simulink model "IEEE39_IBR_FrequencyControl_Fullversion_2021a"  (R2021a)
settings: Solver=VariableStepAuto  StartTime=0.0  StopTime=30  RelTol=1e-3
InitFcn:
  | IEEE39data_FrencyControl_full_Opensource;
undefined symbols (not defined in the file): alpha, c, eps_ps, eps_u, Fref, IBR_data, line, Sbase, t_start_disturbance, t_startcontrol, Vbase
libraries: spsThreePhaseVIMeasurementLib x61, spsThreePhasePISectionLineLib x34, spsControlledVoltageSourceLib x33, spsabctodq0Lib x33, powerlib_extras x27, spsPLL3phLib x26, spsGroundLib x22, spsThreePhaseSeriesRLCBranchLib x22, spsThreePhaseParallelRLCLoadLib x19, pid_lib x14, spsMeanLib x11, spsdq0toabcLib x11
(part 1 of 5)
settings Model: SimulationMode=accelerator  Creator=wangxy  LastModifiedBy=wangxy
settings DebuggingCC: UnconnectedInputMsg=none  UnconnectedOutputMsg=none  UnconnectedLineMsg=none
settings ModelReferenceCC: EnableRefExpFcnMdlSchedulingChecks=off
settings RTWCC: Description=Generic Real-Time Target  GPUComputeCapability=5.0  DLArmComputeVersion=20.02.1

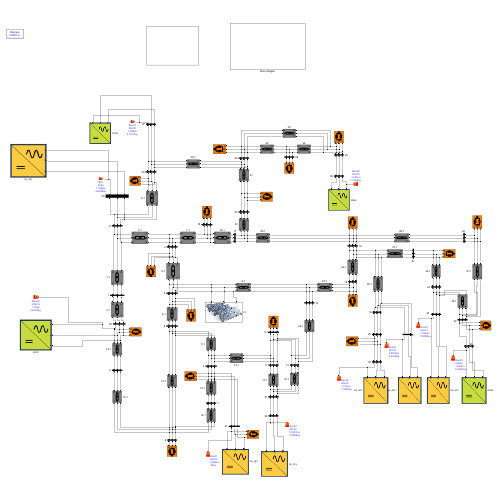
[thumbnail: Simulink's stored preview of the top-level diagram]
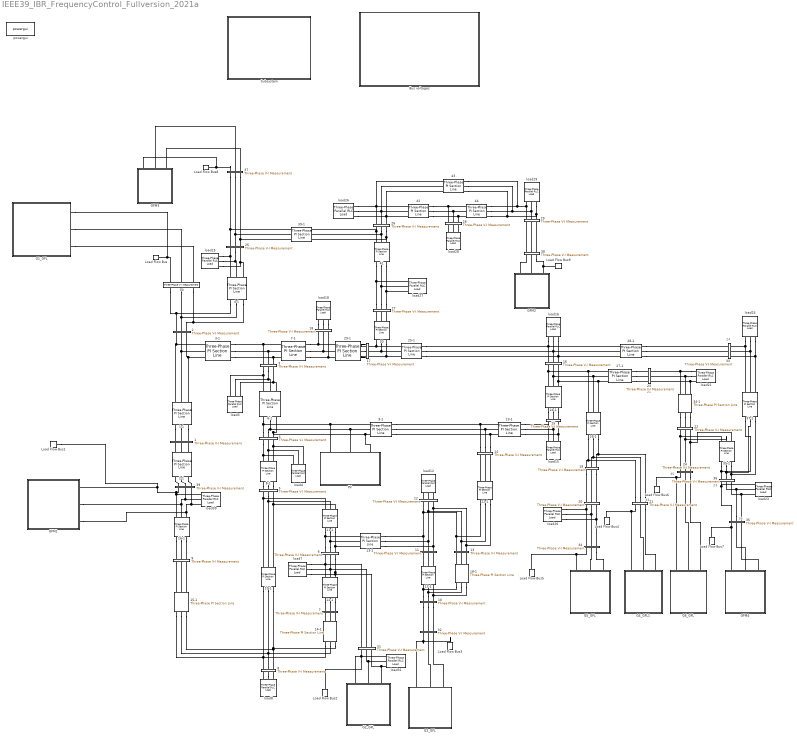
== system IEEE39_IBR_FrequencyControl_Fullversion_2021a ==
  note: 33
  note: 24
  note: 23
  note: 36
  note: 35
  note: 21
  " 30" : spsThreePhasePISectionLineLib/Three-Phase PI Section Line  LConnTagsString=a|b|c  RConnTagsString=A|B|C  Length=1  Frequency=60  Resistances="[line(30,3)  3*line(30,3)]"  Inductances="[line(30,4)  3*line(30,4)]"  Capacitances="[line(30,5)  line(30,5)/3]"
  1 : spsThreePhaseVIMeasurementLib/Three-Phase V-I Measurement  VoltageMeasurement=phase-to-phase  SetLabelV=on  LabelV=Vabc_1  Vpu=off  VpuLL=on  CurrentMeasurement=no  SetLabelI=on  LabelI=Iabc_B2  Ipu=off  Pbase=100e6  Vbase=Bus(1,2)*1e3  OutputType=Complex  PhasorSimulation=off  PSBequivalent=0
  1-1 : spsThreePhasePISectionLineLib/Three-Phase PI Section Line  LConnTagsString=a|b|c  RConnTagsString=A|B|C  Length=1  Frequency=60  Resistances="[line(1,3)  3*line(1,3)]"  Inductances="[line(1,4)  3*line(1,4)]"  Capacitances="[line(1,5)  line(1,5)/3]"
  10 : spsThreePhaseVIMeasurementLib/Three-Phase V-I Measurement  VoltageMeasurement=phase-to-phase  SetLabelV=on  LabelV=Vabc_10  Vpu=off  VpuLL=on  CurrentMeasurement=no  SetLabelI=on  LabelI=Iabc_B2  Ipu=off  Pbase=100e6  Vbase=Bus(10,2)*1e3  OutputType=Complex  PhasorSimulation=off  PSBequivalent=0
  10-1 : spsThreePhasePISectionLineLib/Three-Phase PI Section Line  LConnTagsString=a|b|c  RConnTagsString=A|B|C  Length=1  Frequency=60  Resistances="[line(10,3)  3*line(10,3)]"  Inductances="[line(10,4)  3*line(10,4)]"  Capacitances="[line(10,5)  line(10,5)/3]"
  11 : spsThreePhaseVIMeasurementLib/Three-Phase V-I Measurement  VoltageMeasurement=phase-to-phase  SetLabelV=on  LabelV=Vabc_11  Vpu=off  VpuLL=on  CurrentMeasurement=no  SetLabelI=on  LabelI=Iabc_B2  Ipu=off  Pbase=100e6  Vbase=Bus(11,2)*1e3  OutputType=Complex  PhasorSimulation=off  PSBequivalent=0
  11-1 : spsThreePhasePISectionLineLib/Three-Phase PI Section Line  LConnTagsString=a|b|c  RConnTagsString=A|B|C  Length=1  Frequency=60  Resistances="[line(11,3)  3*line(11,3)]"  Inductances="[line(11,4)  3*line(11,4)]"  Capacitances="[line(11,5)   line(11,5)/3]"
  12 : spsThreePhaseVIMeasurementLib/Three-Phase V-I Measurement  VoltageMeasurement=phase-to-phase  SetLabelV=on  LabelV=Vabc_12  Vpu=off  VpuLL=on  CurrentMeasurement=no  SetLabelI=on  LabelI=Iabc_B2  Ipu=off  Pbase=100e6  Vbase=Bus(12,2)*1e3  OutputType=Complex  PhasorSimulation=off  PSBequivalent=0
  12-1 : spsThreePhasePISectionLineLib/Three-Phase PI Section Line  LConnTagsString=a|b|c  RConnTagsString=A|B|C  Length=1  Frequency=60  Resistances="[line(12,3)  3*line(12,3)]"  Inductances="[line(12,4)  3*line(12,4)]"  Capacitances="[line(12,5)   line(12,5)/3]"
  13 : spsThreePhaseVIMeasurementLib/Three-Phase V-I Measurement  VoltageMeasurement=phase-to-phase  SetLabelV=on  LabelV=Vabc_13  Vpu=off  VpuLL=on  CurrentMeasurement=no  SetLabelI=on  LabelI=Iabc_B2  Ipu=off  Pbase=100e6  Vbase=Bus(13,2)*1e3  OutputType=Complex  PhasorSimulation=off  PSBequivalent=0
  13-1 : spsThreePhasePISectionLineLib/Three-Phase PI Section Line  LConnTagsString=a|b|c  RConnTagsString=A|B|C  Length=1  Frequency=60  Resistances=[line(13,3) 3*line(13,3)]  Inductances="[line(13,4)  3*line(13,4)]"  Capacitances="[line(13,5)  line(13,5)/3]"
  14 : spsThreePhaseVIMeasurementLib/Three-Phase V-I Measurement  VoltageMeasurement=phase-to-phase  SetLabelV=on  LabelV=Vabc_14  Vpu=off  VpuLL=on  CurrentMeasurement=no  SetLabelI=on  LabelI=Iabc_B2  Ipu=off  Pbase=100e6  Vbase=Bus(14,2)*1e3  OutputType=Complex  PhasorSimulation=off  PSBequivalent=0
  14-1 : spsThreePhasePISectionLineLib/Three-Phase PI Section Line  LConnTagsString=a|b|c  RConnTagsString=A|B|C  Length=1  Frequency=60  Resistances=[ line(14,3) 3*line(14,3)]  Inductances="[ line(14,4)  3*line(14,4)]"  Capacitances="[line(14,5)   line(14,5)/3]"
  15 : spsThreePhaseVIMeasurementLib/Three-Phase V-I Measurement  VoltageMeasurement=phase-to-phase  SetLabelV=on  LabelV=Vabc_15  Vpu=off  VpuLL=on  CurrentMeasurement=no  SetLabelI=on  LabelI=Iabc_B2  Ipu=off  Pbase=100e6  Vbase=Bus(15,2)*1e3  OutputType=Complex  PhasorSimulation=off  PSBequivalent=0
  15-1 : spsThreePhasePISectionLineLib/Three-Phase PI Section Line  LConnTagsString=a|b|c  RConnTagsString=A|B|C  Length=1  Frequency=60  Resistances="[line(15,3)  3*line(15,3)]"  Inductances="[line(15,4)  3*line(15,4)]"  Capacitances="[line(15,5)   line(15,5)/5]"
  16 : spsThreePhaseVIMeasurementLib/Three-Phase V-I Measurement  VoltageMeasurement=phase-to-phase  SetLabelV=on  LabelV=Vabc_16  Vpu=off  VpuLL=on  CurrentMeasurement=no  SetLabelI=on  LabelI=Iabc_B2  Ipu=off  Pbase=100e6  Vbase=Bus(16,2)*1e3  OutputType=Complex  PhasorSimulation=off  PSBequivalent=0
  16-1 : spsThreePhasePISectionLineLib/Three-Phase PI Section Line  LConnTagsString=a|b|c  RConnTagsString=A|B|C  Length=1  Frequency=60  Resistances="[line(8,3)  3*line(8,3)]"  Inductances="[line(8,4)  3*line(8,4)]"  Capacitances="[line(8,5)   line(8,5)/3]"
  17 : spsThreePhaseVIMeasurementLib/Three-Phase V-I Measurement  VoltageMeasurement=phase-to-phase  SetLabelV=on  LabelV=Vabc_17  Vpu=off  VpuLL=on  CurrentMeasurement=no  SetLabelI=on  LabelI=Iabc_B2  Ipu=off  Pbase=100e6  Vbase=Bus(17,2)*1e3  OutputType=Complex  PhasorSimulation=off  PSBequivalent=0
  17-1 : spsThreePhasePISectionLineLib/Three-Phase PI Section Line  LConnTagsString=a|b|c  RConnTagsString=A|B|C  Length=1  Frequency=60  Resistances="[line(17,3)  3*line(17,3)]"  Inductances="[line(17,4)  3*line(17,4)]"  Capacitances="[line(17,5)   line(17,5)/3]"
  18 : spsThreePhaseVIMeasurementLib/Three-Phase V-I Measurement  VoltageMeasurement=phase-to-phase  SetLabelV=on  LabelV=Vabc_18  Vpu=off  VpuLL=on  CurrentMeasurement=no  SetLabelI=on  LabelI=Iabc_B2  Ipu=off  Pbase=100e6  Vbase=Bus(18,2)*1e3  OutputType=Complex  PhasorSimulation=off  PSBequivalent=0
  18-1 : spsThreePhasePISectionLineLib/Three-Phase PI Section Line  LConnTagsString=a|b|c  RConnTagsString=A|B|C  Length=1  Frequency=60  Resistances="[line(18,3)  3*line(18,3)]"  Inductances="[line(18,4)  3*line(18,4)]"  Capacitances="[line(18,5)   line(18,5)/3]"
  19 : spsThreePhaseVIMeasurementLib/Three-Phase V-I Measurement  VoltageMeasurement=phase-to-phase  SetLabelV=on  LabelV=Vabc_19  Vpu=off  VpuLL=on  CurrentMeasurement=no  SetLabelI=on  LabelI=Iabc_B2  Ipu=off  Pbase=100e6  Vbase=Bus(19,2)*1e3  OutputType=Complex  PhasorSimulation=off  PSBequivalent=0
  2 : spsThreePhaseVIMeasurementLib/Three-Phase V-I Measurement  VoltageMeasurement=phase-to-phase  SetLabelV=on  LabelV=Vabc_2  Vpu=off  VpuLL=on  CurrentMeasurement=no  SetLabelI=on  LabelI=Iabc_B2  Ipu=off  Pbase=100e6  Vbase=Bus(2,2)*1e3  OutputType=Complex  PhasorSimulation=off  PSBequivalent=0
  2-1 : spsThreePhasePISectionLineLib/Three-Phase PI Section Line  LConnTagsString=a|b|c  RConnTagsString=A|B|C  Length=1  Frequency=60  Resistances="[line(2,3)  3*line(2,3)]"  Inductances="[line(2,4)  3*line(2,4)]"  Capacitances="[line(2,5)   line(2,5)/3]"
  20 : spsThreePhaseVIMeasurementLib/Three-Phase V-I Measurement  VoltageMeasurement=phase-to-phase  SetLabelV=on  LabelV=Vabc_20  Vpu=off  VpuLL=on  CurrentMeasurement=no  SetLabelI=on  LabelI=Iabc_B2  Ipu=off  Pbase=100e6  Vbase=Bus(20,2)*1e3  OutputType=Complex  PhasorSimulation=off  PSBequivalent=0
  21 : spsThreePhaseVIMeasurementLib/Three-Phase V-I Measurement  VoltageMeasurement=phase-to-phase  SetLabelV=on  LabelV=Vabc_33  Vpu=off  VpuLL=on  CurrentMeasurement=no  SetLabelI=on  LabelI=Iabc_B2  Ipu=off  Pbase=100e6  Vbase=Bus(33,2)*1e3  OutputType=Complex  PhasorSimulation=off  PSBequivalent=0
  22 : spsThreePhaseVIMeasurementLib/Three-Phase V-I Measurement  VoltageMeasurement=phase-to-phase  SetLabelV=on  LabelV=Vabc_22  Vpu=off  VpuLL=on  CurrentMeasurement=no  SetLabelI=on  LabelI=Iabc_B2  Ipu=off  Pbase=100e6  Vbase=Bus(22,2)*1e3  OutputType=Complex  PhasorSimulation=off  PSBequivalent=0
  22-1 : spsThreePhasePISectionLineLib/Three-Phase PI Section Line  LConnTagsString=a|b|c  RConnTagsString=A|B|C  Length=1  Frequency=60  Resistances="[line(22,3)  3*line(22,3)]"  Inductances="[line(22,4)  3*line(22,4)]"  Capacitances="[line(22,5)   line(22,5)/3]"
  23 : spsThreePhaseVIMeasurementLib/Three-Phase V-I Measurement  VoltageMeasurement=phase-to-phase  SetLabelV=on  LabelV=Vabc_21  Vpu=off  VpuLL=on  CurrentMeasurement=no  SetLabelI=on  LabelI=Iabc_B2  Ipu=off  Pbase=100e6  Vbase=Bus(21,2)*1e3  OutputType=Complex  PhasorSimulation=off  PSBequivalent=0
  23-1 : spsThreePhasePISectionLineLib/Three-Phase PI Section Line  LConnTagsString=a|b|c  RConnTagsString=A|B|C  Length=1  Frequency=60  Resistances="[line(23,3)  3*line(23,3)]"  Inductances="[line(23,4)  3*line(23,4)]"  Capacitances="[line(23,5)   line(23,5)/3]"
  24 : spsThreePhaseVIMeasurementLib/Three-Phase V-I Measurement  VoltageMeasurement=phase-to-phase  SetLabelV=on  LabelV=Vabc_35  Vpu=off  VpuLL=on  CurrentMeasurement=no  SetLabelI=on  LabelI=Iabc_B2  Ipu=off  Pbase=100e6  Vbase=Bus(35,2)*1e3  OutputType=Complex  PhasorSimulation=off  PSBequivalent=0
  24-1 : spsThreePhasePISectionLineLib/Three-Phase PI Section Line  LConnTagsString=a|b|c  RConnTagsString=A|B|C  Length=1  Frequency=60  Resistances="[line(24,3)  3*line(24,3)]"  Inductances="[line(24,4)  3*line(24,4)]"  Capacitances="[line(24,5)   line(24,5)/3]"
  25 : spsThreePhaseVIMeasurementLib/Three-Phase V-I Measurement  VoltageMeasurement=phase-to-phase  SetLabelV=on  LabelV=Vabc_25  Vpu=off  VpuLL=on  CurrentMeasurement=no  SetLabelI=on  LabelI=Iabc_B2  Ipu=off  Pbase=100e6  Vbase=Bus(25,2)*1e3  OutputType=Complex  PhasorSimulation=off  PSBequivalent=0
  25-1 : spsThreePhasePISectionLineLib/Three-Phase PI Section Line  LConnTagsString=a|b|c  RConnTagsString=A|B|C  Length=1  Frequency=60  Resistances="[ line(25,3)  3*line(25,3)]"  Inductances="[ line(25,4)  3*line(25,4)]"  Capacitances="[line(25,5)  line(25,5)/3]"
  26 : spsThreePhaseVIMeasurementLib/Three-Phase V-I Measurement  VoltageMeasurement=phase-to-phase  SetLabelV=on  LabelV=Vabc_26  Vpu=off  VpuLL=on  CurrentMeasurement=no  SetLabelI=on  LabelI=Iabc_B2  Ipu=off  Pbase=100e6  Vbase=Bus(26,2)*1e3  OutputType=Complex  PhasorSimulation=off  PSBequivalent=0
  26-1 : spsThreePhasePISectionLineLib/Three-Phase PI Section Line  LConnTagsString=a|b|c  RConnTagsString=A|B|C  Length=1  Frequency=60  Resistances="[line(26,3)   3*line(26,3)]"  Inductances="[line(26,4)  3*line(26,4)]"  Capacitances="[line(26,5)   line(26,5)/3]"
  27 : spsThreePhaseVIMeasurementLib/Three-Phase V-I Measurement  VoltageMeasurement=phase-to-phase  SetLabelV=on  LabelV=Vabc_27  Vpu=off  VpuLL=on  CurrentMeasurement=no  SetLabelI=on  LabelI=Iabc_B2  Ipu=off  Pbase=100e6  Vbase=Bus(27,2)*1e3  OutputType=Complex  PhasorSimulation=off  PSBequivalent=0
  27-1 : spsThreePhasePISectionLineLib/Three-Phase PI Section Line  LConnTagsString=a|b|c  RConnTagsString=A|B|C  Length=1  Frequency=60  Resistances="[line(27,3)  3*line(27,3)]"  Inductances="[line(27,4)  3*line(27,4)]"  Capacitances="[line(27,5)   line(27,5)/3]"
  28 : spsThreePhaseVIMeasurementLib/Three-Phase V-I Measurement  VoltageMeasurement=phase-to-phase  SetLabelV=on  LabelV=Vabc_28  Vpu=off  VpuLL=on  CurrentMeasurement=no  SetLabelI=on  LabelI=Iabc_B2  Ipu=off  Pbase=100e6  Vbase=Bus(28,2)*1e3  OutputType=Complex  PhasorSimulation=off  PSBequivalent=0
  28-1 : spsThreePhasePISectionLineLib/Three-Phase PI Section Line  LConnTagsString=a|b|c  RConnTagsString=A|B|C  Length=1  Frequency=60  Resistances=[line(28,3) 3*line(28,3) ]  Inductances="[line(28,4)  3*line(28,4)]"  Capacitances="[line(28,5)   line(28,5)/3]"
  29 : spsThreePhaseVIMeasurementLib/Three-Phase V-I Measurement  VoltageMeasurement=phase-to-phase  SetLabelV=on  LabelV=Vabc_29  Vpu=off  VpuLL=on  CurrentMeasurement=no  SetLabelI=on  LabelI=Iabc_B2  Ipu=off  Pbase=100e6  Vbase=Bus(29,2)*1e3  OutputType=Complex  PhasorSimulation=off  PSBequivalent=0
  29-1 : spsThreePhasePISectionLineLib/Three-Phase PI Section Line  LConnTagsString=a|b|c  RConnTagsString=A|B|C  Length=1  Frequency=60  Resistances=[ line(29,3) 3*line(29,3)]  Inductances="[ line(29,4)  3*line(29,4)]"  Capacitances="[line(29,5)    line(29,5)/3]"
  3 : spsThreePhaseVIMeasurementLib/Three-Phase V-I Measurement  VoltageMeasurement=phase-to-phase  SetLabelV=on  LabelV=Vabc_3  Vpu=off  VpuLL=on  CurrentMeasurement=yes  SetLabelI=on  LabelI=Iabc_B3  Ipu=off  Pbase=100e6  Vbase=Bus(3,2)*1e3  OutputType=Complex  PhasorSimulation=off  PSBequivalent=0
  3-1 : spsThreePhasePISectionLineLib/Three-Phase PI Section Line  LConnTagsString=a|b|c  RConnTagsString=A|B|C  Length=1  Frequency=60  Resistances=[line(3,3) 3*line(3,3)]  Inductances="[line(3,4)  3*line(3,4)]"  Capacitances="[line(3,5)   line(3,5)/3]"
  30 : spsThreePhaseVIMeasurementLib/Three-Phase V-I Measurement  VoltageMeasurement=phase-to-ground  SetLabelV=on  LabelV=Vabc_30  Vpu=off  VpuLL=off  CurrentMeasurement=no  SetLabelI=on  LabelI=Iabc_B2  Ipu=off  Pbase=100e6  Vbase=Bus(30,2)*1e3  OutputType=Complex  PhasorSimulation=off  PSBequivalent=0
  31 : spsThreePhaseVIMeasurementLib/Three-Phase V-I Measurement  VoltageMeasurement=phase-to-phase  SetLabelV=on  LabelV=Vabc_31  Vpu=off  VpuLL=on  CurrentMeasurement=no  SetLabelI=on  LabelI=Iabc_B2  Ipu=off  Pbase=100e6  Vbase=Bus(31,2)*1e3  OutputType=Complex  PhasorSimulation=off  PSBequivalent=0
  32 : spsThreePhaseVIMeasurementLib/Three-Phase V-I Measurement  VoltageMeasurement=phase-to-phase  SetLabelV=on  LabelV=Vabc_32  Vpu=off  VpuLL=on  CurrentMeasurement=no  SetLabelI=on  LabelI=Iabc_B2  Ipu=off  Pbase=100e6  Vbase=Bus(32,2)*1e3  OutputType=Complex  PhasorSimulation=off  PSBequivalent=0
  33 : spsThreePhaseVIMeasurementLib/Three-Phase V-I Measurement  VoltageMeasurement=phase-to-phase  SetLabelV=on  LabelV=Vabc_24  Vpu=off  VpuLL=on  CurrentMeasurement=no  SetLabelI=on  LabelI=Iabc_B2  Ipu=off  Pbase=100e6  Vbase=Bus(24,2)*1e3  OutputType=Complex  PhasorSimulation=off  PSBequivalent=0
  34 : spsThreePhaseVIMeasurementLib/Three-Phase V-I Measurement  VoltageMeasurement=phase-to-phase  SetLabelV=on  LabelV=Vabc_34  Vpu=off  VpuLL=on  CurrentMeasurement=no  SetLabelI=on  LabelI=Iabc_B2  Ipu=off  Pbase=100e6  Vbase=Bus(34,2)*1e3  OutputType=Complex  PhasorSimulation=off  PSBequivalent=0
  34-1 : spsThreePhasePISectionLineLib/Three-Phase PI Section Line  LConnTagsString=a|b|c  RConnTagsString=A|B|C  Length=1  Frequency=60  Resistances="[line(34,3)  3*line(34,3) ]"  Inductances="[line(34,4)  3*line(34,4)]"  Capacitances="[line(34,5)   line(34,5)/3]"
  35 : spsThreePhaseVIMeasurementLib/Three-Phase V-I Measurement  VoltageMeasurement=phase-to-phase  SetLabelV=on  LabelV=Vabc_36  Vpu=off  VpuLL=on  CurrentMeasurement=no  SetLabelI=on  LabelI=Iabc_B2  Ipu=off  Pbase=100e6  Vbase=Bus(36,2)*1e3  OutputType=Complex  PhasorSimulation=off  PSBequivalent=0
  35-1 : spsThreePhasePISectionLineLib/Three-Phase PI Section Line  LConnTagsString=a|b|c  RConnTagsString=A|B|C  Length=1  Frequency=60  Resistances="[line(35,3)  3*line(35,3)]"  Inductances="[line(35,4)  3*line(35,4)]"  Capacitances="[line(35,5)   line(35,5)/3]"
  36 : spsThreePhaseVIMeasurementLib/Three-Phase V-I Measurement  VoltageMeasurement=phase-to-phase  SetLabelV=on  LabelV=Vabc_23  Vpu=off  VpuLL=on  CurrentMeasurement=no  SetLabelI=on  LabelI=Iabc_B2  Ipu=off  Pbase=100e6  Vbase=Bus(23,2)*1e3  OutputType=Complex  PhasorSimulation=off  PSBequivalent=0
  37 : spsThreePhaseVIMeasurementLib/Three-Phase V-I Measurement  VoltageMeasurement=phase-to-phase  SetLabelV=on  LabelV=Vabc_37  Vpu=off  VpuLL=on  CurrentMeasurement=no  SetLabelI=on  LabelI=Iabc_B2  Ipu=off  Pbase=100e6  Vbase=Bus(37,2)*1e3  OutputType=Complex  PhasorSimulation=off  PSBequivalent=0
  37-1 : spsThreePhasePISectionLineLib/Three-Phase PI Section Line  LConnTagsString=a|b|c  RConnTagsString=A|B|C  Length=1  Frequency=60  Resistances="[line(37,3)  3*line(37,3) ]"  Inductances="[line(37,4)  3*line(37,4)]"  Capacitances="[line(37,5)   line(37,5)/3]"
  38 : spsThreePhaseVIMeasurementLib/Three-Phase V-I Measurement  VoltageMeasurement=phase-to-phase  SetLabelV=on  LabelV=Vabc_38  Vpu=off  VpuLL=on  CurrentMeasurement=no  SetLabelI=off  LabelI=Iabc_B2  Ipu=off  Pbase=100e6  Vbase=Bus(38,2)*1e3  OutputType=Complex  PhasorSimulation=off  PSBequivalent=0
  39 : spsThreePhaseVIMeasurementLib/Three-Phase V-I Measurement  VoltageMeasurement=phase-to-phase  SetLabelV=on  LabelV=Vabc_39  Vpu=off  VpuLL=on  CurrentMeasurement=yes  SetLabelI=on  LabelI=Iabc_B2  Ipu=off  Pbase=100e6  Vbase=Bus(39,2)*1e3  OutputType=Complex  PhasorSimulation=off  PSBequivalent=0
  39-1 : spsThreePhasePISectionLineLib/Three-Phase PI Section Line  LConnTagsString=a|b|c  RConnTagsString=A|B|C  Length=1  Frequency=60  Resistances=[ line(39,3) 3* line(39,3)]  Inductances="[ line(39,4)  3*line(39,4)]"  Capacitances="[line(39,5)  line(39,5)/3]"
  4 : spsThreePhaseVIMeasurementLib/Three-Phase V-I Measurement  VoltageMeasurement=phase-to-phase  SetLabelV=on  LabelV=Vabc_4  Vpu=off  VpuLL=on  CurrentMeasurement=yes  SetLabelI=on  LabelI=Iabc_B4  Ipu=off  Pbase=100e6  Vbase=Bus(4,2)*1e3  OutputType=Complex  PhasorSimulation=off  PSBequivalent=0
  4-1 : spsThreePhasePISectionLineLib/Three-Phase PI Section Line  LConnTagsString=a|b|c  RConnTagsString=A|B|C  Length=1  Frequency=60  Resistances="[line(4,3)  3*line(4,3)]"  Inductances="[line(4,4)  3*line(4,4)]"  Capacitances="[line(4,5)   line(4,5)/3]"
  41 : spsThreePhasePISectionLineLib/Three-Phase PI Section Line  LConnTagsString=a|b|c  RConnTagsString=A|B|C  Length=1  Frequency=60  Resistances="[ line(41,3)  3*line(41,3)]"  Inductances="[ line(41,4)  3*line(41,4)]"  Capacitances="[line(41,5)    line(41,5)/3]"
  42 : spsThreePhasePISectionLineLib/Three-Phase PI Section Line  LConnTagsString=a|b|c  RConnTagsString=A|B|C  Length=1  Frequency=60  Resistances="[ line(42,3)   3*line(42,3)]"  Inductances="[ line(42,4)   3*line(42,4)]"  Capacitances="[line(42,5)    line(42,5)/3]"
  43 : spsThreePhasePISectionLineLib/Three-Phase PI Section Line  LConnTagsString=a|b|c  RConnTagsString=A|B|C  Length=1  Frequency=60  Resistances="[ line(43,3)  3* line(43,3) ]"  Inductances="[ line(43,4)   3*line(43,4)]"  Capacitances="[line(43,5)   line(43,5)/3]"
  44 : spsThreePhasePISectionLineLib/Three-Phase PI Section Line  LConnTagsString=a|b|c  RConnTagsString=A|B|C  Length=1  Frequency=60  Resistances="[ line(44,3)  3* line(44,3)]"  Inductances="[ line(44,4)  3* line(44,4)]"  Capacitances="[line(44,5)   line(44,5)/3]"
  5 : spsThreePhaseVIMeasurementLib/Three-Phase V-I Measurement  VoltageMeasurement=phase-to-phase  SetLabelV=on  LabelV=Vabc_5  Vpu=off  VpuLL=on  CurrentMeasurement=no  SetLabelI=on  LabelI=Iabc_B2  Ipu=off  Pbase=100e6  Vbase=Bus(5,2)*1e3  OutputType=Complex  PhasorSimulation=off  PSBequivalent=0
  6 : spsThreePhaseVIMeasurementLib/Three-Phase V-I Measurement  VoltageMeasurement=phase-to-phase  SetLabelV=on  LabelV=Vabc_6  Vpu=off  VpuLL=on  CurrentMeasurement=no  SetLabelI=on  LabelI=Iabc_B2  Ipu=off  Pbase=100e6  Vbase=Bus(6,2)*1e3  OutputType=Complex  PhasorSimulation=off  PSBequivalent=0
  6-1 : spsThreePhasePISectionLineLib/Three-Phase PI Section Line  LConnTagsString=a|b|c  RConnTagsString=A|B|C  Length=1  Frequency=60  Resistances="[line(6,3)    3*line(6,3) ]"  Inductances="[line(6,4)   3*line(6,4)]"  Capacitances="[line(6,5)   line(6,5)/3]"
  7 : spsThreePhaseVIMeasurementLib/Three-Phase V-I Measurement  VoltageMeasurement=phase-to-phase  SetLabelV=on  LabelV=Vabc_7  Vpu=off  VpuLL=on  CurrentMeasurement=no  SetLabelI=on  LabelI=Iabc_B2  Ipu=off  Pbase=100e6  Vbase=Bus(8,2)*1e3  OutputType=Complex  PhasorSimulation=off  PSBequivalent=0
  7-1 : spsThreePhasePISectionLineLib/Three-Phase PI Section Line  LConnTagsString=a|b|c  RConnTagsString=A|B|C  Length=1  Frequency=60  Resistances="[line(7,3)  3*line(7,3)]"  Inductances="[line(7,4)  3*line(7,4)]"  Capacitances="[line(7,5)   line(7,5)/3]"
  8 : spsThreePhaseVIMeasurementLib/Three-Phase V-I Measurement  VoltageMeasurement=phase-to-phase  SetLabelV=on  LabelV=Vabc_8  Vpu=off  VpuLL=on  CurrentMeasurement=no  SetLabelI=on  LabelI=Iabc_B2  Ipu=off  Pbase=100e6  Vbase=Bus(8,2)*1e3  OutputType=Complex  PhasorSimulation=off  PSBequivalent=0
  8-1 : spsThreePhasePISectionLineLib/Three-Phase PI Section Line  LConnTagsString=a|b|c  RConnTagsString=A|B|C  Length=1  Frequency=60  Resistances="[line(8,3)  3*line(8,3) ]"  Inductances="[line(8,4)  3*line(8,4)]"  Capacitances="[line(8,5)   line(8,5)/3]"
  9 : spsThreePhaseVIMeasurementLib/Three-Phase V-I Measurement  VoltageMeasurement=phase-to-phase  SetLabelV=on  LabelV=Vabc_9  Vpu=off  VpuLL=on  CurrentMeasurement=no  SetLabelI=on  LabelI=Iabc_B2  Ipu=off  Pbase=100e6  Vbase=Bus(9,2)*1e3  OutputType=Complex  PhasorSimulation=off  PSBequivalent=0
  9-1 : spsThreePhasePISectionLineLib/Three-Phase PI Section Line  LConnTagsString=a|b|c  RConnTagsString=A|B|C  Length=1  Frequency=60  Resistances="[ line(9,3)  3*line(9,3) ]"  Inductances="[ line(9,4)  3*line(9,4)]"  Capacitances="[line(9,5)   line(9,5)/3]"
  Bus voltages : Subsystem
  G1_GFL : Subsystem
      mask Display: image('GFL.png');
  G2_GFL : Subsystem
      mask Display: image('GFL.png');
  G3_GFL : Subsystem
      mask Display: image('GFL.png');
  G4_GFL1 : Subsystem
      mask Display: image('GFL.png');
  G5_GFL : Subsystem
      mask Display: image('GFL.png');
  G6_GFL : Subsystem
      mask Display: image('GFL.png');
  GFM1 : Subsystem
      mask Display: image('GFM.png');
  GFM2 : Subsystem
      mask Display: image('GFM.png');
  GFM3 : Subsystem
      mask Display: image('GFM.png');
  GFM4 : Subsystem
      mask Display: image('GFM.png');
  Load Flow Bus : spsLoadFlowBusLib/Load Flow Bus  LConnTagsString=a  Phases=single  Connectors=on one side  ID=B30  Vbase=22e3  Vref=1.0475  Vangle=0  VLF=1.048  VLFb=1  VLFc=1  angleLF=-3.646  angleLFb=0  angleLFc=0
      settings: AttributesFormatString=%<ID>\n%<Vbase>\n%<VLF>pu\n%<angleLF>deg.
  Load Flow Bus1 : spsLoadFlowBusLib/Load Flow Bus  LConnTagsString=a  Phases=single  Connectors=on one side  ID=Bus39  Vbase=345e3  Vref=1.03  Vangle=0  VLF=1.03  VLFb=1  VLFc=1  angleLF=19.62  angleLFb=0  angleLFc=0
      settings: AttributesFormatString=%<ID>\n%<Vbase>V\n%<VLF>pu\n%<angleLF>deg.
  Load Flow Bus2 : spsLoadFlowBusLib/Load Flow Bus  LConnTagsString=a  Phases=single  Connectors=on one side  ID=Bus31  Vbase=22e3  Vref=0.9820  Vangle=0  VLF=0.982  VLFb=1  VLFc=1  angleLF=0  angleLFb=0  angleLFc=0
      settings: AttributesFormatString=%<ID>\n%<Vbase>V\n%<VLF>pu\n%<angleLF>deg.
  Load Flow Bus3 : spsLoadFlowBusLib/Load Flow Bus  LConnTagsString=a  Phases=single  Connectors=on one side  ID=Bus32  Vbase=22e3  Vref=0.9831  Vangle=0  VLF=0.9831  VLFb=1  VLFc=1  angleLF=2.466  angleLFb=0  angleLFc=0
      settings: AttributesFormatString=%<ID>\n%<Vbase>V\n%<VLF>pu\n%<angleLF>deg.
  Load Flow Bus4 : spsLoadFlowBusLib/Load Flow Bus  LConnTagsString=a  Phases=single  Connectors=on one side  ID=Bus33  Vbase=22e3  Vref=0.9972  Vangle=0  VLF=0.9972  VLFb=1  VLFc=1  angleLF=4.423  angleLFb=0  angleLFc=0
      settings: AttributesFormatString=%<ID>\n%<Vbase>V\n%<VLF>pu\n%<angleLF>deg.
  Load Flow Bus5 : spsLoadFlowBusLib/Load Flow Bus  LConnTagsString=a  Phases=single  Connectors=on one side  ID=Bus34  Vbase=22e3  Vref=1.0123  Vangle=0  VLF=1.012  VLFb=1  VLFc=1  angleLF=3.398  angleLFb=0  angleLFc=0
      settings: AttributesFormatString=%<ID>\n%<Vbase>V\n%<VLF>pu\n%<angleLF>deg.
  Load Flow Bus6 : spsLoadFlowBusLib/Load Flow Bus  LConnTagsString=a  Phases=single  Connectors=on one side  ID=Bus35  Vbase=22e3  Vref=1.0493  Vangle=0  VLF=1.049  VLFb=1  VLFc=1  angleLF=5.698  angleLFb=0  angleLFc=0
      settings: AttributesFormatString=%<ID>\n%<Vbase>V\n%<VLF>pu\n%<angleLF>deg.
  Load Flow Bus7 : spsLoadFlowBusLib/Load Flow Bus  LConnTagsString=a  Phases=single  Connectors=on one side  ID=Bus36  Vbase=22e3  Vref=1.0635  Vangle=0  VLF=1.063  VLFb=1  VLFc=1  angleLF=8.494  angleLFb=0  angleLFc=0
      settings: AttributesFormatString=%<ID>\n%<Vbase>V\n%<VLF>pu\n%<angleLF>deg.
  Load Flow Bus8 : spsLoadFlowBusLib/Load Flow Bus  LConnTagsString=a  Phases=single  Connectors=on one side  ID=Bus37  Vbase=22e3  Vref=1.0278  Vangle=0  VLF=1.028  VLFb=1  VLFc=1  angleLF=2.181  angleLFb=0  angleLFc=0
      settings: AttributesFormatString=%<ID>\n%<Vbase>V\n%<VLF>pu\n%<angleLF>deg.
  Load Flow Bus9 : spsLoadFlowBusLib/Load Flow Bus  LConnTagsString=a  Phases=single  Connectors=on one side  ID=Bus38  Vbase=22e3  Vref=1.0265  Vangle=0  VLF=1.027  VLFb=1  VLFc=1  angleLF=7.784  angleLFb=0  angleLFc=0
      settings: AttributesFormatString=%<ID>\n%<Vbase>V\n%<VLF>pu\n%<angleLF>deg.
  PV : Subsystem
      mask Display: image('PV.jpg');
  Subsystem : Subsystem
  load12 : spsThreePhaseParallelRLCLoadLib/Three-Phase Parallel RLC Load  LConnTagsString=A|B|C  Configuration=Y (grounded)  NominalVoltage=(345e3)*0.939625  Vabc=[1e3 1e3 1e3]  Vabcp=[1e3 1e3 1e3]  NominalFrequency=60  UnbalancedPower=off  ActivePower=8.53e6  InductivePower=88e6  CapacitivePower=0  Pabc=[10e3 9e3 11e3]  QLabc=[100 90 110]  QCabc=[100 90 110]  Pabcp=[10e3 9e3 11e3]  QLabcp=[100 90 110]  QCabcp=[100 90 110]  Measurements=None  LoadType=constant PQ
  load15 : spsThreePhaseParallelRLCLoadLib/Three-Phase Parallel RLC Load  LConnTagsString=A|B|C  Configuration=Y (grounded)  NominalVoltage=(345e3)*0.969586  Vabc=[1e3 1e3 1e3]  Vabcp=[1e3 1e3 1e3]  NominalFrequency=60  UnbalancedPower=off  ActivePower=320e6  InductivePower=153e6  CapacitivePower=0  Pabc=[10e3 9e3 11e3]  QLabc=[100 90 110]  QCabc=[100 90 110]  Pabcp=[10e3 9e3 11e3]  QLabcp=[100 90 110]  QCabcp=[100 90 110]  Measurements=None  LoadType=constant PQ
  load16 : spsThreePhaseParallelRLCLoadLib/Three-Phase Parallel RLC Load  LConnTagsString=A|B|C  Configuration=Y (grounded)  NominalVoltage=(345e3)*0.988678  Vabc=[1e3 1e3 1e3]  Vabcp=[1e3 1e3 1e3]  NominalFrequency=60  UnbalancedPower=off  ActivePower=329e6  InductivePower=32.3e6  CapacitivePower=0  Pabc=[10e3 9e3 11e3]  QLabc=[100 90 110]  QCabc=[100 90 110]  Pabcp=[10e3 9e3 11e3]  QLabcp=[100 90 110]  QCabcp=[100 90 110]  Measurements=None  LoadType=constant PQ
  load18 : spsThreePhaseParallelRLCLoadLib/Three-Phase Parallel RLC Load  LConnTagsString=A|B|C  Configuration=Y (grounded)  NominalVoltage=(345e3)*0.991132  Vabc=[1e3 1e3 1e3]  Vabcp=[1e3 1e3 1e3]  NominalFrequency=60  UnbalancedPower=off  ActivePower=158e6  InductivePower=30e6  CapacitivePower=0  Pabc=[10e3 9e3 11e3]  QLabc=[100 90 110]  QCabc=[100 90 110]  Pabcp=[10e3 9e3 11e3]  QLabcp=[100 90 110]  QCabcp=[100 90 110]  Measurements=None  LoadType=constant PQ
  load20 : spsThreePhaseParallelRLCLoadLib/Three-Phase Parallel RLC Load  LConnTagsString=A|B|C  Configuration=Y (grounded)  NominalVoltage=(345e3)*0.987086  Vabc=[1e3 1e3 1e3]  Vabcp=[1e3 1e3 1e3]  NominalFrequency=60  UnbalancedPower=off  ActivePower=628e6  InductivePower=103e6  CapacitivePower=0  Pabc=[10e3 9e3 11e3]  QLabc=[100 90 110]  QCabc=[100 90 110]  Pabcp=[10e3 9e3 11e3]  QLabcp=[100 90 110]  QCabcp=[100 90 110]  Measurements=None  LoadType=constant PQ
  load21 : spsThreePhaseParallelRLCLoadLib/Three-Phase Parallel RLC Load  LConnTagsString=A|B|C  Configuration=Y (grounded)  NominalVoltage=(345e3)*0.995503  Vabc=[1e3 1e3 1e3]  Vabcp=[1e3 1e3 1e3]  NominalFrequency=60  UnbalancedPower=off  ActivePower=274e6  InductivePower=115e6  CapacitivePower=0  Pabc=[10e3 9e3 11e3]  QLabc=[100 90 110]  QCabc=[100 90 110]  Pabcp=[10e3 9e3 11e3]  QLabcp=[100 90 110]  QCabcp=[100 90 110]  Measurements=None  LoadType=constant PQ
  load23 : spsThreePhaseParallelRLCLoadLib/Three-Phase Parallel RLC Load  LConnTagsString=A|B|C  Configuration=Y (grounded)  NominalVoltage=(345e3)*1.02041  Vabc=[1e3 1e3 1e3]  Vabcp=[1e3 1e3 1e3]  NominalFrequency=60  UnbalancedPower=off  ActivePower=247.5e6  InductivePower=84.6e6  CapacitivePower=0  Pabc=[10e3 9e3 11e3]  QLabc=[100 90 110]  QCabc=[100 90 110]  Pabcp=[10e3 9e3 11e3]  QLabcp=[100 90 110]  QCabcp=[100 90 110]  Measurements=None  LoadType=constant PQ
  load24 : spsThreePhaseParallelRLCLoadLib/Three-Phase Parallel RLC Load  LConnTagsString=A|B|C  Configuration=Y (grounded)  NominalVoltage=(345e3)*0.996934  Vabc=[1e3 1e3 1e3]  Vabcp=[1e3 1e3 1e3]  NominalFrequency=60  UnbalancedPower=off  ActivePower=308.6e6  InductivePower=0  CapacitivePower=9.2e6  Pabc=[10e3 9e3 11e3]  QLabc=[100 90 110]  QCabc=[100 90 110]  Pabcp=[10e3 9e3 11e3]  QLabcp=[100 90 110]  QCabcp=[100 90 110]  Measurements=None  LoadType=constant PQ
  load25 : spsThreePhaseParallelRLCLoadLib/Three-Phase Parallel RLC Load  LConnTagsString=A|B|C  Configuration=Y (grounded)  NominalVoltage=(345e3)*1.0284  Vabc=[1e3 1e3 1e3]  Vabcp=[1e3 1e3 1e3]  NominalFrequency=60  UnbalancedPower=off  ActivePower=224e6  InductivePower=47.2e6  CapacitivePower=0  Pabc=[10e3 9e3 11e3]  QLabc=[100 90 110]  QCabc=[100 90 110]  Pabcp=[10e3 9e3 11e3]  QLabcp=[100 90 110]  QCabcp=[100 90 110]  Measurements=None  LoadType=constant PQ
  load26 : spsThreePhaseParallelRLCLoadLib/Three-Phase Parallel RLC Load  LConnTagsString=A|B|C  Configuration=Y (grounded)  NominalVoltage=(345e3)*1.01809  Vabc=[1e3 1e3 1e3]  Vabcp=[1e3 1e3 1e3]  NominalFrequency=60  UnbalancedPower=off  ActivePower=139e6  InductivePower=17e6  CapacitivePower=0  Pabc=[10e3 9e3 11e3]  QLabc=[100 90 110]  QCabc=[100 90 110]  Pabcp=[10e3 9e3 11e3]  QLabcp=[100 90 110]  QCabcp=[100 90 110]  Measurements=None  LoadType=constant PQ
  load27 : spsThreePhaseParallelRLCLoadLib/Three-Phase Parallel RLC Load  LConnTagsString=A|B|C  Configuration=Y (grounded)  NominalVoltage=(345e3)*1.00029  Vabc=[1e3 1e3 1e3]  Vabcp=[1e3 1e3 1e3]  NominalFrequency=60  UnbalancedPower=off  ActivePower=281e6  InductivePower=75.5e6  CapacitivePower=0  Pabc=[10e3 9e3 11e3]  QLabc=[100 90 110]  QCabc=[100 90 110]  Pabcp=[10e3 9e3 11e3]  QLabcp=[100 90 110]  QCabcp=[100 90 110]  Measurements=None  LoadType=constant PQ
  load28 : spsThreePhaseParallelRLCLoadLib/Three-Phase Parallel RLC Load  LConnTagsString=A|B|C  Configuration=Y (grounded)  NominalVoltage=(345e3)*1.01937  Vabc=[1e3 1e3 1e3]  Vabcp=[1e3 1e3 1e3]  NominalFrequency=60  UnbalancedPower=off  ActivePower=206e6  InductivePower=276e6  CapacitivePower=0  Pabc=[10e3 9e3 11e3]  QLabc=[100 90 110]  QCabc=[100 90 110]  Pabcp=[10e3 9e3 11e3]  QLabcp=[100 90 110]  QCabcp=[100 90 110]  Measurements=None  LoadType=constant PQ
  load29 : spsThreePhaseParallelRLCLoadLib/Three-Phase Parallel RLC Load  LConnTagsString=A|B|C  Configuration=Y (grounded)  NominalVoltage=(345e3)*1.02077  Vabc=[1e3 1e3 1e3]  Vabcp=[1e3 1e3 1e3]  NominalFrequency=60  UnbalancedPower=off  ActivePower=283.5e6  InductivePower=26.9e6  CapacitivePower=0  Pabc=[10e3 9e3 11e3]  QLabc=[100 90 110]  QCabc=[100 90 110]  Pabcp=[10e3 9e3 11e3]  QLabcp=[100 90 110]  QCabcp=[100 90 110]  Measurements=None  LoadType=constant PQ
  load3 : spsThreePhaseParallelRLCLoadLib/Three-Phase Parallel RLC Load  LConnTagsString=A|B|C  Configuration=Y (grounded)  NominalVoltage=(345e3)*0.992094  Vabc=[1e3 1e3 1e3]  Vabcp=[1e3 1e3 1e3]  NominalFrequency=60  UnbalancedPower=off  ActivePower=322e6  InductivePower=2.4e6  CapacitivePower=0  Pabc=[10e3 9e3 11e3]  QLabc=[100 90 110]  QCabc=[100 90 110]  Pabcp=[10e3 9e3 11e3]  QLabcp=[100 90 110]  QCabcp=[100 90 110]  Measurements=None  LoadType=constant PQ
  load31 : spsThreePhaseParallelRLCLoadLib/Three-Phase Parallel RLC Load  LConnTagsString=A|B|C  Configuration=Y (grounded)  NominalVoltage=(345e3)*0.982  Vabc=[1e3 1e3 1e3]  Vabcp=[1e3 1e3 1e3]  NominalFrequency=60  UnbalancedPower=off  ActivePower=92e6  InductivePower=46e6  CapacitivePower=0  Pabc=[10e3 9e3 11e3]  QLabc=[100 90 110]  QCabc=[100 90 110]  Pabcp=[10e3 9e3 11e3]  QLabcp=[100 90 110]  QCabcp=[100 90 110]  Measurements=None  LoadType=constant PQ
  load39 : spsThreePhaseParallelRLCLoadLib/Three-Phase Parallel RLC Load  LConnTagsString=A|B|C  Configuration=Y (grounded)  NominalVoltage=(345e3)*1.05  Vabc=[1e3 1e3 1e3]  Vabcp=[1e3 1e3 1e3]  NominalFrequency=60  UnbalancedPower=off  ActivePower=500e6  InductivePower=300e6  CapacitivePower=0  Pabc=[10e3 9e3 11e3]  QLabc=[100 90 110]  QCabc=[100 90 110]  Pabcp=[10e3 9e3 11e3]  QLabcp=[100 90 110]  QCabcp=[100 90 110]  Measurements=None  LoadType=constant PQ
  load4 : spsThreePhaseParallelRLCLoadLib/Three-Phase Parallel RLC Load  LConnTagsString=A|B|C  Configuration=Y (grounded)  NominalVoltage=(345e3)*1  Vabc=[1e3 1e3 1e3]  Vabcp=[1e3 1e3 1e3]  NominalFrequency=60  UnbalancedPower=off  ActivePower=500e6  InductivePower=184e6  CapacitivePower=0  Pabc=[10e3 9e3 11e3]  QLabc=[100 90 110]  QCabc=[100 90 110]  Pabcp=[10e3 9e3 11e3]  QLabcp=[100 90 110]  QCabcp=[100 90 110]  Measurements=None  LoadType=constant PQ
  load7 : spsThreePhaseParallelRLCLoadLib/Three-Phase Parallel RLC Load  LConnTagsString=A|B|C  Configuration=Y (grounded)  NominalVoltage=(345e3)*0.956463  Vabc=[1e3 1e3 1e3]  Vabcp=[1e3 1e3 1e3]  NominalFrequency=60  UnbalancedPower=off  ActivePower=233e6  InductivePower=84e6  CapacitivePower=0  Pabc=[10e3 9e3 11e3]  QLabc=[100 90 110]  QCabc=[100 90 110]  Pabcp=[10e3 9e3 11e3]  QLabcp=[100 90 110]  QCabcp=[100 90 110]  Measurements=None  LoadType=constant PQ
  load8 : spsThreePhaseParallelRLCLoadLib/Three-Phase Parallel RLC Load  LConnTagsString=A|B|C  Configuration=Y (grounded)  NominalVoltage=(345e3)*0.954036  Vabc=[1e3 1e3 1e3]  Vabcp=[1e3 1e3 1e3]  NominalFrequency=60  UnbalancedPower=off  ActivePower=522e6  InductivePower=176e6  CapacitivePower=0  Pabc=[10e3 9e3 11e3]  QLabc=[100 90 110]  QCabc=[100 90 110]  Pabcp=[10e3 9e3 11e3]  QLabcp=[100 90 110]  QCabcp=[100 90 110]  Measurements=None  LoadType=constant PQ
  powergui : spspowerguiLib/powergui  Priority=2  SimulationMode=Discrete  SampleTime=1e-4  frequency=60  Iterations=50  frequencyindice=60  Pbase=100e6  ErrMax=0.0001  UnitsV=kV  UnitsW=MW  buscounter=0  FunctionMessages=off  echomessages=off  EnableUseOfTLC=off  CurrentSourceSwitches=off  DisableSnubberDevices=off  DisableRonSwitches=off  DisableVfSwitches=off  DisplayEquations=off  AutomaticDiscreteSolvers=off  SolverType=Tustin  Interpol=off  ExternalGateDelay=off  methode=off  Ts=0  x0status=blocks  SPID=off  SwTol=0  HookPort=off  NonlinearTolerance=1e-4  nMaxIteration=100  ContinueOnMaxIteration=off  RestoreLinks=warning  ResistiveCurrentMeasurement=off  Frange=logspace(0,3,50)  Ylog=off  Xlog=off  ShowGrid=off  save=off  variable=ZData  structure=0  ZoomFFT=on  StartTime=0.0  cycles=1  DisplayStyle=1  fundamental=60  FreqAxis=off  MaxFrequency=1000  frequencyindicesteady=1  RmsSteady=1  display=off
  connections:
  load31/LConn2 -- G2_GFL/RConn2 -- 31/RConn2
  24-1/LConn1 -- 16/LConn1 -- 26-1/LConn1 -- 27-1/RConn1
  26/LConn3 -- 43/RConn3 -- 42/RConn3 -- load26/LConn3
  15-1/RConn2 -- 8/LConn2 -- 14-1/RConn2 -- 10-1/RConn2
  7-1/LConn2 -- 29-1/RConn2 -- 18/RConn2
  load31/LConn3 -- 31/RConn3 -- G2_GFL/RConn3
  load29/LConn1 -- 29/RConn1 -- 44/LConn1 -- 43/LConn1
  load26/LConn1 -- 43/RConn1 -- 42/RConn1 -- 26/LConn1
  21/LConn1 -- G4_GFL1/RConn1 -- Load Flow Bus4/LConn1
  25/LConn2 -- 37/RConn2 -- 39-1/RConn2
  2/RConn2 -- 3-1/RConn2 -- 1-1/LConn2
  3/RConn1 -- 6-1/LConn1 -- load3/LConn1
  load39/LConn2 -- 16-1/LConn2 -- GFM1/RConn2 -- 39/RConn2
  Load Flow Bus1/LConn1 -- 16-1/LConn1 -- load39/LConn1 -- 39/RConn1 -- GFM1/RConn1
  44/LConn2 -- 43/LConn2 -- 29/RConn2 -- load29/LConn2
  10/LConn1 -- 18-1/RConn1 -- 17-1/RConn1
  36/LConn3 -- 35-1/RConn3 -- 37-1/RConn3
  29/RConn3 -- load29/LConn3 -- 44/LConn3 -- 43/LConn3
  7-1/LConn3 -- 29-1/RConn3 -- 18/RConn3
  4-1/RConn3 -- 30/RConn3 -- 2/LConn3
  36/LConn2 -- 35-1/RConn2 -- 37-1/RConn2
  3/RConn3 -- 6-1/LConn3 -- load3/LConn3
  Load Flow Bus5/LConn1 -- 34/RConn1 -- G5_GFL/RConn1
  3/LConn3 -- 7-1/RConn3 -- 3-1/LConn3
  16/LConn2 -- 26-1/LConn2 -- 27-1/RConn2 -- 24-1/LConn2
  load21/LConn2 -- 34-1/LConn2 -- 23/RConn2
  28/RConn3 -- 42/LConn3 -- 44/RConn3
  15/RConn3 -- 23-1/LConn3 -- load15/LConn3
  6/LConn3 -- 13-1/LConn3 -- 11-1/RConn3
  15/RConn2 -- 23-1/LConn2 -- load15/LConn2
  26/RConn1 -- 41/RConn1 -- 39-1/LConn1
  2/RConn3 -- 3-1/RConn3 -- 1-1/LConn3
  3/RConn2 -- 6-1/LConn2 -- load3/LConn2
  15-1/RConn3 -- 8/LConn3 -- 14-1/RConn3 -- 10-1/RConn3
  16/LConn3 -- 26-1/LConn3 -- 27-1/RConn3 -- 24-1/LConn3
  6/LConn2 -- 13-1/LConn2 -- 11-1/RConn2
  16/RConn3 -- 28-1/RConn3 -- 25-1/LConn3 -- load16/LConn3
  10/LConn3 -- 18-1/RConn3 -- 17-1/RConn3
  5/RConn1 -- 11-1/LConn1 -- 10-1/LConn1
  10/LConn2 -- 18-1/RConn2 -- 17-1/RConn2
  24/RConn1 -- Load Flow Bus6/LConn1 -- G6_GFL/RConn1
  16/RConn1 -- 28-1/RConn1 -- 25-1/LConn1 -- load16/LConn1
  37/RConn3 -- 25/LConn3 -- 39-1/RConn3
  12/RConn3 -- 22-1/RConn3 -- 13/LConn3 -- 13-1/RConn3 -- 11/LConn3
  load25/LConn2 -- 4-1/LConn2 -- 25/RConn2
  3/LConn1 -- 7-1/RConn1 -- 3-1/LConn1
  4/LConn3 -- PV/RConn3 -- 9-1/RConn3 -- 6-1/RConn3
  28/RConn1 -- 42/LConn1 -- 44/RConn1
  33/RConn2 -- 37-1/LConn2 -- load24/LConn2
  28/RConn2 -- 42/LConn2 -- 44/RConn2
  27/LConn2 -- 41/LConn2 -- load27/LConn2
  30/LConn1 -- G1_GFL/RConn1 -- Load Flow Bus/LConn1
  37/LConn1 -- GFM3/RConn1 -- Load Flow Bus8/LConn1
  35/RConn1 -- GFM4/RConn1 -- Load Flow Bus7/LConn1
  14/RConn3 -- 23-1/RConn3 -- 9-1/LConn3
  load25/LConn1 -- 4-1/LConn1 -- 25/RConn1
  14/RConn2 -- 23-1/RConn2 -- 9-1/LConn2
  load26/LConn2 -- 43/RConn2 -- 42/RConn2 -- 26/LConn2
  12/RConn1 -- 22-1/RConn1 -- 13/LConn1 -- 13-1/RConn1 -- 11/LConn1
  27/LConn3 -- 41/LConn3 -- load27/LConn3
  26/RConn2 -- 41/RConn2 -- 39-1/LConn2
  5/RConn3 -- 11-1/LConn3 -- 10-1/LConn3
  17/LConn2 -- 25-1/RConn2 -- " 30"/RConn2
  4/RConn3 -- load4/LConn3 -- 8-1/LConn3
  15/RConn1 -- 23-1/LConn1 -- load15/LConn1
  16/RConn2 -- 28-1/RConn2 -- 25-1/LConn2 -- load16/LConn2
  25/RConn3 -- 4-1/LConn3 -- load25/LConn3
  36/LConn1 -- 35-1/RConn1 -- 37-1/RConn1
  4-1/RConn1 -- 30/RConn1 -- 2/LConn1
  5/RConn2 -- 11-1/LConn2 -- 10-1/LConn2
  load21/LConn3 -- 34-1/LConn3 -- 23/RConn3
  17/LConn3 -- 25-1/RConn3 -- " 30"/RConn3
  4/LConn2 -- 9-1/RConn2 -- PV/RConn2 -- 6-1/RConn2
  6/LConn1 -- 13-1/LConn1 -- 11-1/RConn1
  27/LConn1 -- 41/LConn1 -- load27/LConn1
  17/LConn1 -- 25-1/RConn1 -- " 30"/RConn1
  25/LConn1 -- 37/RConn1 -- 39-1/RConn1
  load4/LConn2 -- 4/RConn2 -- 8-1/LConn2
  2/RConn1 -- 3-1/RConn1 -- 1-1/LConn1
  4-1/RConn2 -- 30/RConn2 -- 2/LConn2
  14/RConn1 -- 23-1/RConn1 -- 9-1/LConn1
  4/LConn1 -- 9-1/RConn1 -- PV/RConn1 -- 6-1/RConn1
  3-1/LConn2 -- 3/LConn2 -- 7-1/RConn2
  load21/LConn1 -- 34-1/LConn1 -- 23/RConn1
  33/RConn1 -- 37-1/LConn1 -- load24/LConn1
  31/RConn1 -- G2_GFL/RConn1 -- Load Flow Bus2/LConn1 -- load31/LConn1
  8/LConn1 -- 14-1/RConn1 -- 10-1/RConn1 -- 15-1/RConn1
  7-1/LConn1 -- 29-1/RConn1 -- 18/RConn1
  33/RConn3 -- 37-1/LConn3 -- load24/LConn3
  4/RConn1 -- load4/LConn1 -- 8-1/LConn1
  26/RConn3 -- 39-1/LConn3 -- 41/RConn3
  38/RConn3 -- GFM2/RConn3 -- Load Flow Bus9/LConn1
  12/RConn2 -- 22-1/RConn2 -- 13/LConn2 -- 13-1/RConn2 -- 11/LConn2
  20/RConn1 -- 34/LConn1 -- load20/LConn1
  21/RConn3 -- 19/LConn3 -- 26-1/RConn3
  10/RConn3 -- 32/LConn3
  load8/LConn1 -- 8/RConn1
  34-1/RConn2 -- 22/LConn2
  22-1/LConn3 -- 14/LConn3
  12/LConn2 -- load12/LConn2
  " 30"/LConn2 -- 27/RConn2
  14-1/LConn3 -- 7/LConn3
  24-1/RConn3 -- 15/LConn3
  8-1/RConn1 -- 5/LConn1
  load8/LConn3 -- 8/RConn3
  load28/LConn1 -- 28/LConn1
  27-1/LConn1 -- 23/LConn1
  12-1/RConn3 -- 7/RConn3
  " 30"/LConn3 -- 27/RConn3
  29-1/LConn3 -- 17/RConn3
  29-1/LConn2 -- 17/RConn2
  34-1/RConn3 -- 22/LConn3
  20/LConn2 -- 19/RConn2
  load7/LConn3 -- 12-1/LConn3 -- 6/RConn3 -- 31/LConn3
  22/RConn1 -- 35-1/LConn1 -- 24/LConn1
  15-1/LConn1 -- 9/RConn1
  2-1/LConn1 -- 1/RConn1
  24-1/RConn1 -- 15/LConn1
  35/LConn2 -- 36/RConn2 -- load23/LConn2
  17-1/LConn3 -- 11/RConn3
  18-1/LConn3 -- 13/RConn3
  19/RConn3 -- 20/LConn3
  16-1/RConn2 -- 9/LConn2
  1-1/RConn2 -- 1/LConn2
  2-1/LConn2 -- 1/RConn2
  14-1/LConn2 -- 7/LConn2
  17-1/LConn1 -- 11/RConn1
  15-1/LConn2 -- 9/RConn2
  20/RConn3 -- 34/LConn3 -- load20/LConn3
  load23/LConn3 -- 36/RConn3 -- 35/LConn3
  10/RConn2 -- 32/LConn2
  21/RConn2 -- 19/LConn2 -- 26-1/RConn2
  22-1/LConn1 -- 14/LConn1
  2-1/LConn3 -- 1/RConn3
  28-1/LConn2 -- 33/LConn2
  12-1/RConn1 -- 7/RConn1
  20/RConn2 -- 34/LConn2 -- load20/LConn2
  22/RConn3 -- 35-1/LConn3 -- 24/LConn3
  " 30"/LConn1 -- 27/RConn1
  16-1/RConn3 -- 9/LConn3
  27-1/LConn3 -- 23/LConn3
  load18/LConn2 -- 18/LConn2
  6/RConn1 -- 12-1/LConn1 -- 31/LConn1 -- load7/LConn1
  12/LConn1 -- load12/LConn1
  2-1/RConn1 -- 39/LConn1
  load18/LConn1 -- 18/LConn1
  29-1/LConn1 -- 17/RConn1
  19/RConn1 -- 20/LConn1
  14-1/LConn1 -- 7/LConn1
  load28/LConn2 -- 28/LConn2
  1-1/RConn1 -- 1/LConn1
  16-1/RConn1 -- 9/LConn1
  load18/LConn3 -- 18/LConn3
  15-1/LConn3 -- 9/RConn3
  load28/LConn3 -- 28/LConn3
  8/RConn2 -- load8/LConn2
  17-1/LConn2 -- 11/RConn2
  18-1/LConn1 -- 13/RConn1
  28-1/LConn3 -- 33/LConn3
  1-1/RConn3 -- 1/LConn3
  8-1/RConn2 -- 5/LConn2
  27-1/LConn2 -- 23/LConn2
  2-1/RConn3 -- 39/LConn3
  12/LConn3 -- load12/LConn3
  28-1/LConn1 -- 33/LConn1
  2-1/RConn2 -- 39/LConn2
  12-1/RConn2 -- 7/RConn2
  36/RConn1 -- 35/LConn1 -- load23/LConn1
  8-1/RConn3 -- 5/LConn3
  10/RConn1 -- 32/LConn1
  6/RConn2 -- 12-1/LConn2 -- 31/LConn2 -- load7/LConn2
  21/RConn1 -- 19/LConn1 -- 26-1/RConn1
  22-1/LConn2 -- 14/LConn2
  34-1/RConn1 -- 22/LConn1
  24-1/RConn2 -- 15/LConn2
  18-1/LConn2 -- 13/RConn2
  22/RConn2 -- 35-1/LConn2 -- 24/LConn2
  load39/LConn3 -- GFM1/RConn3 -- 16-1/LConn3 -- 39/RConn3
  38/LConn1 -- 29/LConn1
  38/LConn2 -- 29/LConn2
  38/LConn3 -- 29/LConn3
  GFM2/RConn1 -- 38/RConn1
  GFM2/RConn2 -- 38/RConn2
  37/LConn2 -- GFM3/RConn2
  37/LConn3 -- GFM3/RConn3
  GFM4/RConn2 -- 35/RConn2
  GFM4/RConn3 -- 35/RConn3
  G1_GFL/RConn2 -- 30/LConn2
  G1_GFL/RConn3 -- 30/LConn3
  Load Flow Bus3/LConn1 -- G3_GFL/RConn1 -- 32/RConn1
  G3_GFL/RConn2 -- 32/RConn2
  G3_GFL/RConn3 -- 32/RConn3
  G4_GFL1/RConn2 -- 21/LConn2
  21/LConn3 -- G4_GFL1/RConn3
  G5_GFL/RConn2 -- 34/RConn2
  34/RConn3 -- G5_GFL/RConn3
  G6_GFL/RConn2 -- 24/RConn2
  24/RConn3 -- G6_GFL/RConn3

== system IEEE39_IBR_FrequencyControl_Fullversion_2021a/Bus voltages ==
  V_F_measurements30 : Subsystem
  V_F_measurements31 : Subsystem
  V_F_measurements32 : Subsystem
  V_F_measurements33 : Subsystem
  V_F_measurements34 : Subsystem
  V_F_measurements35 : Subsystem
  V_F_measurements36 : Subsystem
  V_F_measurements37 : Subsystem
  V_F_measurements38 : Subsystem
  V_F_measurements39 : Subsystem
  wires:
  [Vabc_31] -> V_F_measurements31/1(abc)
  [Vabc_32] -> V_F_measurements32/1(abc)
  [Vabc_33] -> V_F_measurements33/1(abc)
  [Vabc_34] -> V_F_measurements34/1(abc)
  [Vabc_35] -> V_F_measurements35/1(abc)
  [Vabc_30] -> V_F_measurements30/1(abc)
  [Vabc_36] -> V_F_measurements36/1(abc)
  [Vabc_37] -> V_F_measurements37/1(abc)
  [Vabc_38] -> V_F_measurements38/1(abc)
  [Vabc_39] -> V_F_measurements39/1(abc)

== system IEEE39_IBR_FrequencyControl_Fullversion_2021a/G1_GFL ==
  D : Constant  Value=IBR_data(1,4)
  Fref : Constant  Value=60
  PV_PQ3 : Subsystem
  Pref3 : Constant  Value=IBR_data(1,6)*Sbase
  Qref3 : Constant  Value=IBR_data(1,7)*Sbase*0
  A : PMIOPort  Side=Right
  B : PMIOPort  Port=2  Side=Right
  C : PMIOPort  Port=3  Side=Right
  wires:
  Qref3/1 -> PV_PQ3/2(Qref)
  Fref/1 -> PV_PQ3/3(Fref)
  D/1 -> PV_PQ3/4(D)
  Pref3/1 -> PV_PQ3/1(Pref)
  connections:
  PV_PQ3/RConn1 -- A/RConn1
  PV_PQ3/RConn2 -- B/RConn1
  PV_PQ3/RConn3 -- C/RConn1

== system IEEE39_IBR_FrequencyControl_Fullversion_2021a/G2_GFL ==
  D : Constant  Value=IBR_data(2,4)
  Fref : Constant  Value=60
  PV_PQ3 : Subsystem
  Pref3 : Constant  Value=IBR_data(2,6)*Sbase
  Qref3 : Constant  Value=IBR_data(2,7)*Sbase
  A : PMIOPort  Side=Right
  B : PMIOPort  Port=2  Side=Right
  C : PMIOPort  Port=3  Side=Right
  wires:
  Pref3/1 -> PV_PQ3/1(Pref)
  Qref3/1 -> PV_PQ3/2(Qref)
  Fref/1 -> PV_PQ3/3(Fref)
  D/1 -> PV_PQ3/4(D)
  connections:
  PV_PQ3/RConn1 -- A/RConn1
  PV_PQ3/RConn2 -- B/RConn1
  PV_PQ3/RConn3 -- C/RConn1

== system IEEE39_IBR_FrequencyControl_Fullversion_2021a/G3_GFL ==
  D : Constant  Value=IBR_data(3,4)
  Fref : Constant  Value=60
  PV_PQ3 : Subsystem
  Pref3 : Constant  Value=IBR_data(3,6)*Sbase
  Qref3 : Constant  Value=IBR_data(3,7)*Sbase
  A : PMIOPort  Side=Right
  B : PMIOPort  Port=2  Side=Right
  C : PMIOPort  Port=3  Side=Right
  wires:
  Pref3/1 -> PV_PQ3/1(Pref)
  Qref3/1 -> PV_PQ3/2(Qref)
  Fref/1 -> PV_PQ3/3(Fref)
  D/1 -> PV_PQ3/4(D)
  connections:
  PV_PQ3/RConn1 -- A/RConn1
  PV_PQ3/RConn2 -- B/RConn1
  PV_PQ3/RConn3 -- C/RConn1

== system IEEE39_IBR_FrequencyControl_Fullversion_2021a/G4_GFL1 ==
  D : Constant  Value=IBR_data(4,4)
  Fref : Constant  Value=60
  PV_PQ3 : Subsystem
  Pref3 : Constant  Value=IBR_data(4,6)*Sbase
  Qref3 : Constant  Value=IBR_data(4,7)*Sbase  VectorParams1D=off
  A : PMIOPort  Side=Right
  B : PMIOPort  Port=2  Side=Right
  C : PMIOPort  Port=3  Side=Right
  wires:
  Pref3/1 -> PV_PQ3/1(Pref)
  Qref3/1 -> PV_PQ3/2(Qref)
  Fref/1 -> PV_PQ3/3(Fref)
  D/1 -> PV_PQ3/4(D)
  connections:
  PV_PQ3/RConn1 -- A/RConn1
  PV_PQ3/RConn2 -- B/RConn1
  PV_PQ3/RConn3 -- C/RConn1

== system IEEE39_IBR_FrequencyControl_Fullversion_2021a/G5_GFL ==
  D : Constant  Value=IBR_data(5,4)
  Fref : Constant  Value=60
  PV_PQ3 : Subsystem
  Pref3 : Constant  Value=IBR_data(5,6)*Sbase
  Qref3 : Constant  Value=IBR_data(5,7)*Sbase
  A : PMIOPort  Side=Right
  B : PMIOPort  Port=2  Side=Right
  C : PMIOPort  Port=3  Side=Right
  wires:
  Pref3/1 -> PV_PQ3/1(Pref)
  Qref3/1 -> PV_PQ3/2(Qref)
  Fref/1 -> PV_PQ3/3(Fref)
  D/1 -> PV_PQ3/4(D)
  connections:
  PV_PQ3/RConn1 -- A/RConn1
  PV_PQ3/RConn2 -- B/RConn1
  PV_PQ3/RConn3 -- C/RConn1

== system IEEE39_IBR_FrequencyControl_Fullversion_2021a/G6_GFL ==
  D : Constant  Value=IBR_data(6,4)
  Fref : Constant  Value=60
  PV_PQ3 : Subsystem
  Pref3 : Constant  Value=IBR_data(6,6)*Sbase
  Qref3 : Constant  Value=IBR_data(6,7)*Sbase
  A : PMIOPort  Side=Right
  B : PMIOPort  Port=2  Side=Right
  C : PMIOPort  Port=3  Side=Right
  wires:
  Pref3/1 -> PV_PQ3/1(Pref)
  Qref3/1 -> PV_PQ3/2(Qref)
  Fref/1 -> PV_PQ3/3(Fref)
  D/1 -> PV_PQ3/4(D)
  connections:
  PV_PQ3/RConn1 -- A/RConn1
  PV_PQ3/RConn2 -- B/RConn1
  PV_PQ3/RConn3 -- C/RConn1

== system IEEE39_IBR_FrequencyControl_Fullversion_2021a/GFM1 ==
  Fref : Constant  Value=Fref
  PV_PQ3 : Subsystem
  Phase : Constant  Value=0
  Pref3 : Constant  Value=IBR_data(10,6)*Sbase
  Vref_LL : Constant  Value=IBR_data(10,8)*Vbase
  a : PMIOPort  Side=Right
  b : PMIOPort  Port=2  Side=Right
  c : PMIOPort  Port=3  Side=Right
  wires:
  Pref3/1 -> PV_PQ3/1(Pref)
  Phase/1 -> PV_PQ3/4(Initial_phase)
  Vref_LL/1 -> PV_PQ3/2(Vref_LL)
  Fref/1 -> PV_PQ3/3(Fref)
  connections:
  a/RConn1 -- PV_PQ3/RConn1
  b/RConn1 -- PV_PQ3/RConn2
  c/RConn1 -- PV_PQ3/RConn3

== system IEEE39_IBR_FrequencyControl_Fullversion_2021a/GFM2 ==
  Fref : Constant  Value=Fref
  PV_PQ3 : Subsystem
  Phase : Constant  Value=0.02
  Pref3 : Constant  Value=IBR_data(9,6)*Sbase
  Vref_LL : Constant  Value=IBR_data(10,8)*Vbase
  a : PMIOPort  Side=Right
  b : PMIOPort  Port=2  Side=Right
  c : PMIOPort  Port=3  Side=Right
  wires:
  Pref3/1 -> PV_PQ3/1(Pref)
  Phase/1 -> PV_PQ3/4(Initial_phase)
  Vref_LL/1 -> PV_PQ3/2(Vref_LL)
  Fref/1 -> PV_PQ3/3(Fref)
  connections:
  a/RConn1 -- PV_PQ3/RConn1
  b/RConn1 -- PV_PQ3/RConn2
  c/RConn1 -- PV_PQ3/RConn3

== system IEEE39_IBR_FrequencyControl_Fullversion_2021a/GFM3 ==
  Fref : Constant  Value=Fref
  PV_PQ3 : Subsystem
  Phase : Constant  Value=0.002
  Pref3 : Constant  Value=IBR_data(8,6)*Sbase
  Vref_LL : Constant  Value=IBR_data(10,8)*Vbase
  a : PMIOPort  Side=Right
  b : PMIOPort  Port=2  Side=Right
  c : PMIOPort  Port=3  Side=Right
  wires:
  Pref3/1 -> PV_PQ3/1(Pref)
  Phase/1 -> PV_PQ3/4(Initial_phase)
  Vref_LL/1 -> PV_PQ3/2(Vref_LL)
  Fref/1 -> PV_PQ3/3(Fref)
  connections:
  a/RConn1 -- PV_PQ3/RConn1
  b/RConn1 -- PV_PQ3/RConn2
  c/RConn1 -- PV_PQ3/RConn3

== system IEEE39_IBR_FrequencyControl_Fullversion_2021a/GFM4 ==
  Fref : Constant  Value=Fref
  PV_PQ3 : Subsystem
  Phase : Constant  Value=-0.01
  Pref3 : Constant  Value=IBR_data(7,6)*Sbase
  Vref_LL : Constant  Value=IBR_data(10,8)*Vbase
  a : PMIOPort  Side=Right
  b : PMIOPort  Port=2  Side=Right
  c : PMIOPort  Port=3  Side=Right
  wires:
  Pref3/1 -> PV_PQ3/1(Pref)
  Phase/1 -> PV_PQ3/4(Initial_phase)
  Vref_LL/1 -> PV_PQ3/2(Vref_LL)
  Fref/1 -> PV_PQ3/3(Fref)
  connections:
  a/RConn1 -- PV_PQ3/RConn1
  b/RConn1 -- PV_PQ3/RConn2
  c/RConn1 -- PV_PQ3/RConn3
